simulink library "courseFollowLookAhead_cl"  (R2022a)
settings: Solver=VariableStepAuto  StartTime=0.0  StopTime=10.0  RelTol=1e-3
undefined symbols (not defined in the file or in its folder): a, pathCtrl
libraries: pathGeometry_ul x3, angleBtw2Vecs_ul x3, tanFrameProjection_ul x2, vectorNormalizer_ul x2
settings Model: Creator=James Reed  LastModifiedBy=adabney
settings SolverCC: AlgebraicLoopSolver=TrustRegion
settings DataIOCC: ReturnWorkspaceOutputs=off
settings DebuggingCC: UnconnectedInputMsg=warning  UnconnectedOutputMsg=warning  UnconnectedLineMsg=warning  SFMachineParentedDataDiag=warning  ArithmeticOperatorsInVariantConditions=warning
settings SFSimCC: CustomCodeUndefinedFunction=UseInterfaceOnly

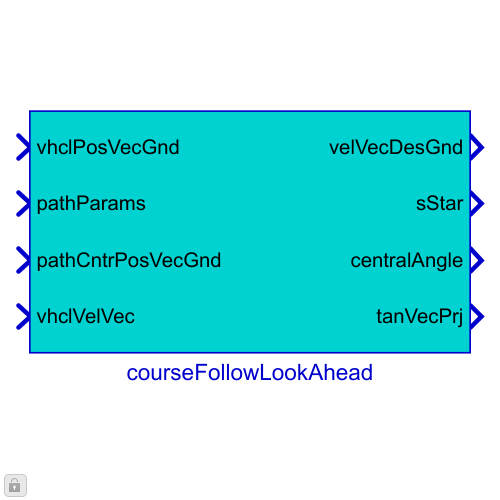
[thumbnail: Simulink's stored preview of the top-level diagram]
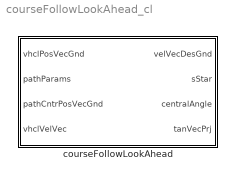
== system courseFollowLookAhead_cl ==
  courseFollowLookAhead : Subsystem

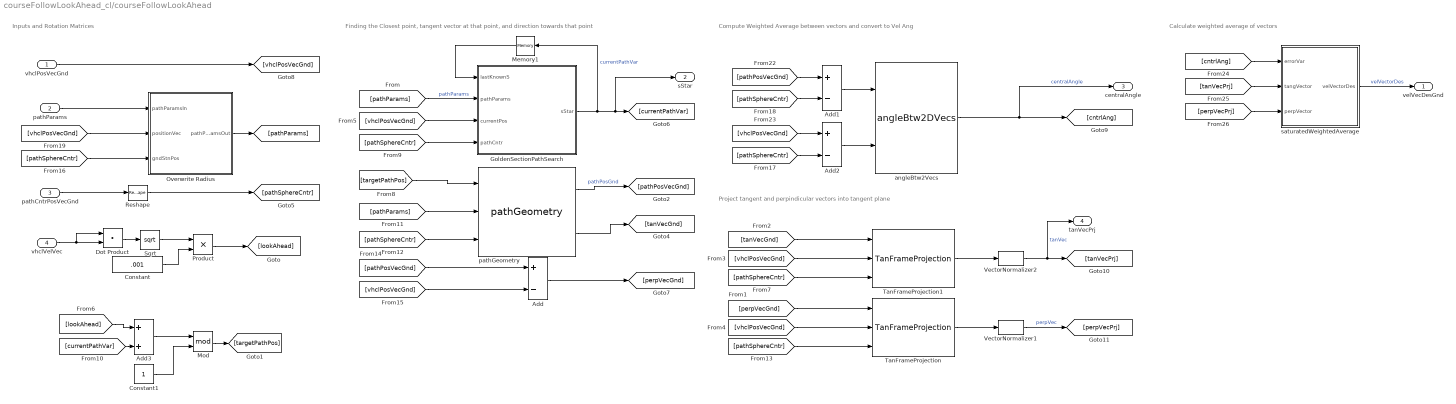
== system courseFollowLookAhead_cl/courseFollowLookAhead ==
  note: Calculate weighted average of vectors
  note: Project tangent and perpindicular vectors into tangent plane
  note: Compute Weighted Average between vectors and convert to Vel Ang
  note: Inputs and Rotation Matrices
  note: Finding the Closest point, tangent vector at that point, and direction towards that point
  "vhclPosVecGnd " : Inport
  pathParams : Inport  Port=2
  pathCntrPosVecGnd : Inport  Port=3
  vhclVelVec : Inport  Port=4
  Add : Sum  Inputs=+-
  Add1 : Sum  Inputs=+-
  Add2 : Sum  Inputs=+-
  Add3 : Sum
  Constant : Constant  Value=.001
  Constant1 : Constant
  Dot Product : DotProduct  OutDataTypeStr=Inherit: Inherit via internal rule
  GoldenSectionPathSearch : Subsystem  TreatAsAtomicUnit=on
  Memory1 : Memory  InitialCondition=pathCtrl.initPathVar.Value
  Mod : Math  Operator=mod
  Overwrite Radius : Subsystem
  Product : Product
  Reshape : Reshape  OutputDimensionality=Column vector (2-D)
  Sqrt : Sqrt
  TanFrameProjection : tanFrameProjection_ul/TanFrameProjection  SystemSampleTime=-1  VariantActivationTime=update diagram  Latency=0  AutoFrameSizeCalculation=off
  TanFrameProjection1 : tanFrameProjection_ul/TanFrameProjection  SystemSampleTime=-1  VariantActivationTime=update diagram  Latency=0  AutoFrameSizeCalculation=off
  VectorNormalizer1 : vectorNormalizer_ul/VectorNormalizer   SystemSampleTime=-1  VariantActivationTime=update diagram  Latency=0  AutoFrameSizeCalculation=off
  VectorNormalizer2 : vectorNormalizer_ul/VectorNormalizer   SystemSampleTime=-1  VariantActivationTime=update diagram  Latency=0  AutoFrameSizeCalculation=off
  angleBtw2Vecs : angleBtw2Vecs_ul/angleBtw2DVecs  SystemSampleTime=-1  VariantActivationTime=update diagram  Latency=0  AutoFrameSizeCalculation=off
  pathGeometry : pathGeometry_ul/pathGeometry  SystemSampleTime=-1  VariantActivationTime=update diagram  Latency=0  AutoFrameSizeCalculation=off
  saturatedWeightedAverage : Subsystem  mask{error_upper_lim=pathCtrl.perpErrorVal.Value}
      mask prompts: error_upper_lim "Value of Error yielding 100% perpendicular"
  velVecDesGnd : Outport  VectorParamsAs1DForOutWhenUnconnected=off
  sStar : Outport  Port=2  VectorParamsAs1DForOutWhenUnconnected=off
  centralAngle : Outport  Port=3  VectorParamsAs1DForOutWhenUnconnected=off
  tanVecPrj : Outport  Port=4
  wires:
  [pathPosVecGnd] -> Add1/1
  VectorNormalizer2/1 -> tanVecPrj/1, [tanVecPrj]  "tanVec"
  [vhclPosVecGnd] -> GoldenSectionPathSearch/3(currentPos)
  "vhclPosVecGnd "/1 -> [vhclPosVecGnd]
  pathGeometry/1 -> [pathPosVecGnd]  "pathPosGnd"
  [pathParams] -> pathGeometry/2
  VectorNormalizer1/1 -> [perpVecPrj]  "perpVec"
  angleBtw2Vecs/1 -> [cntrlAng], centralAngle/1  "centralAngle"
  [vhclPosVecGnd] -> Add2/1
  TanFrameProjection1/1 -> VectorNormalizer2/1
  [pathParams] -> GoldenSectionPathSearch/2(pathParams)  "pathParams"
  GoldenSectionPathSearch/1(sStar) -> Memory1/1, sStar/1, [currentPathVar]  "currentPathVar"
  Memory1/1 -> GoldenSectionPathSearch/1(lastKnownS)
  Add/1 -> [perpVecGnd]
  [vhclPosVecGnd] -> Add/2
  [pathPosVecGnd] -> Add/1
  pathGeometry/2 -> [tanVecGnd]
  TanFrameProjection/1 -> VectorNormalizer1/1
  Overwrite Radius/1(pathParamsOut) -> [pathParams]
  pathCntrPosVecGnd/1 -> Reshape/1
  Reshape/1 -> [pathSphereCntr]
  [pathSphereCntr] -> pathGeometry/3
  [pathSphereCntr] -> GoldenSectionPathSearch/4(pathCntr)
  [pathSphereCntr] -> Add2/2
  [pathSphereCntr] -> Add1/2
  Add1/1 -> angleBtw2Vecs/1
  Add2/1 -> angleBtw2Vecs/2
  [perpVecGnd] -> TanFrameProjection/1
  [tanVecGnd] -> TanFrameProjection1/1
  [vhclPosVecGnd] -> TanFrameProjection1/2
  [vhclPosVecGnd] -> TanFrameProjection/2
  [pathSphereCntr] -> TanFrameProjection1/3
  [pathSphereCntr] -> TanFrameProjection/3
  [cntrlAng] -> saturatedWeightedAverage/1("errorVar ")
  [tanVecPrj] -> saturatedWeightedAverage/2(tangVector)
  [perpVecPrj] -> saturatedWeightedAverage/3("perpVector ")
  saturatedWeightedAverage/1("velVectorDes ") -> velVecDesGnd/1  "velVectorDes"
  vhclVelVec/1 -> Dot Product/1, Dot Product/2
  Dot Product/1 -> Sqrt/1
  Sqrt/1 -> Product/1
  Constant/1 -> Product/2
  Product/1 -> [lookAhead]
  Add3/1 -> Mod/1
  [lookAhead] -> Add3/1
  [currentPathVar] -> Add3/2
  Constant1/1 -> Mod/2
  Mod/1 -> [targetPathPos]
  [targetPathPos] -> pathGeometry/1
  [vhclPosVecGnd] -> Overwrite Radius/2(positionVec)
  [pathSphereCntr] -> Overwrite Radius/3(gndStnPos)
  pathParams/1 -> Overwrite Radius/1(pathParamsIn)

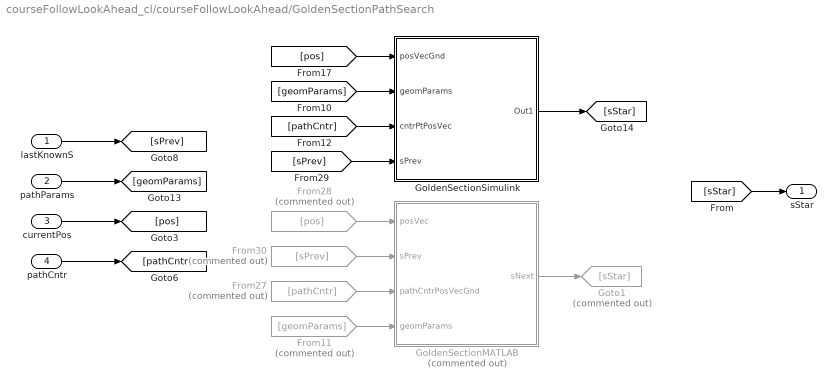
== system courseFollowLookAhead_cl/courseFollowLookAhead/GoldenSectionPathSearch ==
  lastKnownS : Inport
  pathParams : Inport  Port=2
  currentPos : Inport  Port=3
  pathCntr : Inport  Port=4
  From11 : From  Commented=on  GotoTag=geomParams
  From27 : From  Commented=on  GotoTag=pathCntr
  From28 : From  Commented=on  GotoTag=pos
  From30 : From  Commented=on  GotoTag=sPrev
  GoldenSectionMATLAB : MATLAB Function  Commented=on  TreatAsAtomicUnit=on  mask{geomFunc=pathCtrl, searchWidth=0.1, pathVarTol=1e-5}
  GoldenSectionSimulink : Subsystem
  Goto1 : Goto  Commented=on  GotoTag=sStar
  sStar : Outport  InitialOutput=pathCtrl.initPathVar.Value  VectorParamsAs1DForOutWhenUnconnected=off
  wires:
  currentPos/1 -> [pos]
  pathParams/1 -> [geomParams]
  pathCntr/1 -> [pathCntr]
  GoldenSectionMATLAB/1(sNext) -> Goto1/1
  From11/1 -> GoldenSectionMATLAB/4(geomParams)
  From28/1 -> GoldenSectionMATLAB/1(posVec)
  From30/1 -> GoldenSectionMATLAB/2(sPrev)
  From27/1 -> GoldenSectionMATLAB/3(pathCntrPosVecGnd)
  lastKnownS/1 -> [sPrev]
  [sStar] -> sStar/1
  [pos] -> GoldenSectionSimulink/1(posVecGnd)
  [geomParams] -> GoldenSectionSimulink/2(geomParams)
  [pathCntr] -> GoldenSectionSimulink/3(cntrPtPosVec)
  [sPrev] -> GoldenSectionSimulink/4(sPrev)
  GoldenSectionSimulink/1(Out1) -> [sStar]

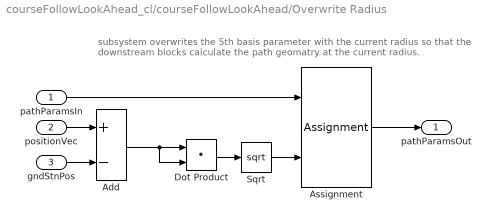
== system courseFollowLookAhead_cl/courseFollowLookAhead/Overwrite Radius ==
  note: subsystem overwrites the 5th basis parameter with the current radius
      | so that the downstream blocks calculate the path geomatry at the current radius.
  pathParamsIn : Inport
  positionVec : Inport  Port=2
  gndStnPos : Inport  Port=3
  Add : Sum  Inputs=+-
  Assignment : Assignment  NumberOfDimensions=2  DiagnosticForDimensions=Warning  IndexOptions=Index vector (dialog),Assign all  Indices=5,5  OutputSizes=1,1
  Dot Product : DotProduct  OutDataTypeStr=Inherit: Inherit via internal rule
  Sqrt : Sqrt
  pathParamsOut : Outport  VectorParamsAs1DForOutWhenUnconnected=off
  wires:
  Add/1 -> Dot Product/2, Dot Product/1
  Dot Product/1 -> Sqrt/1
  Assignment/1 -> pathParamsOut/1
  Sqrt/1 -> Assignment/2
  pathParamsIn/1 -> Assignment/1
  positionVec/1 -> Add/1
  gndStnPos/1 -> Add/2

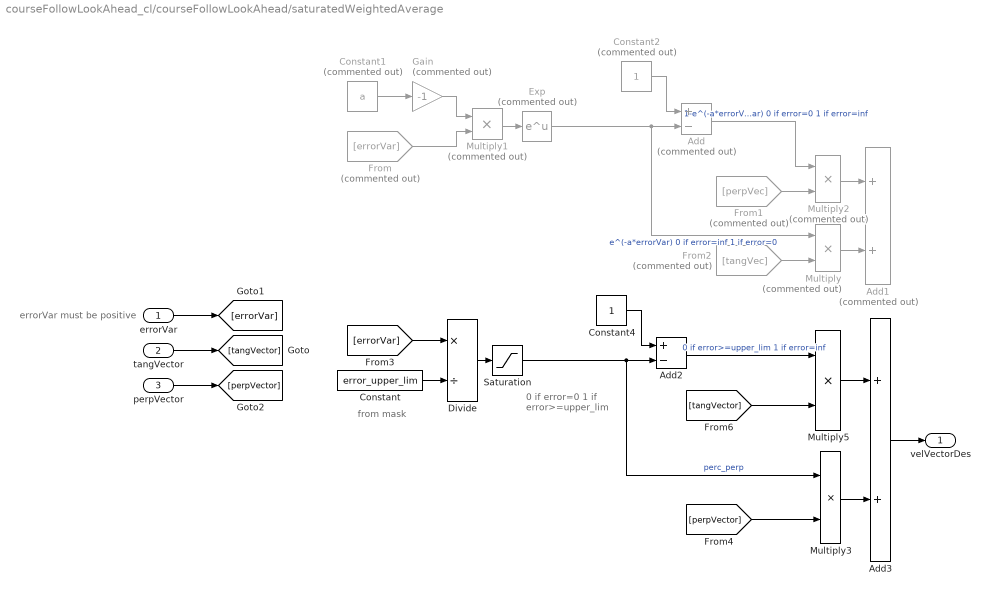
== system courseFollowLookAhead_cl/courseFollowLookAhead/saturatedWeightedAverage ==
  note: errorVar must be positive
  note: from mask
  note: 0 if error=0
      | 1 if error>=upper_lim
  "errorVar " : Inport
  tangVector : Inport  Port=2
  "perpVector " : Inport  Port=3
  Add : Sum  Commented=on  Inputs=+-
  Add1 : Sum  Commented=on
  Add2 : Sum  Inputs=+-
  Add3 : Sum
  Constant : Constant  Value=error_upper_lim
  Constant1 : Constant  Commented=on  Value=a
  Constant2 : Constant  Commented=on
  Constant4 : Constant
  Divide : Product  Inputs=*/
  Exp : Math  Commented=on  SignedPower=on
  From : From  Commented=on  GotoTag=errorVar
  From1 : From  Commented=on  GotoTag=perpVec
  From2 : From  Commented=on  GotoTag=tangVec
  Gain : Gain  Commented=on  Gain=-1
  Multiply : Product  Commented=on
  Multiply1 : Product  Commented=on
  Multiply2 : Product  Commented=on
  Multiply3 : Product
  Multiply5 : Product
  Saturation : Saturate  UpperLimit=1  LowerLimit=0
  "velVectorDes " : Outport  VectorParamsAs1DForOutWhenUnconnected=off
  wires:
  [perpVector] -> Multiply3/2
  [tangVector] -> Multiply5/2
  Divide/1 -> Saturation/1
  Constant/1 -> Divide/2
  [errorVar] -> Divide/1
  Add2/1 -> Multiply5/1  "0 if error>=upper_lim 1 if error=inf"
  Multiply5/1 -> Add3/1
  Multiply3/1 -> Add3/2
  Add3/1 -> "velVectorDes "/1
  Saturation/1 -> Add2/2, Multiply3/1  "perc_perp"
  Constant4/1 -> Add2/1
  From2/1 -> Multiply/2
  From1/1 -> Multiply2/2
  Multiply/1 -> Add1/2
  Multiply2/1 -> Add1/1
  From/1 -> Multiply1/2
  "perpVector "/1 -> [perpVector]
  "errorVar "/1 -> [errorVar]
  Add/1 -> Multiply2/1  "1-e^(-a*errorVar) 0 if error=0 1 if error=inf"
  Constant2/1 -> Add/1
  Exp/1 -> Add/2, Multiply/1  "e^(-a*errorVar) 0 if error=inf 1 if error=0"
  Multiply1/1 -> Exp/1
  Gain/1 -> Multiply1/1
  Constant1/1 -> Gain/1
  tangVector/1 -> [tangVector]

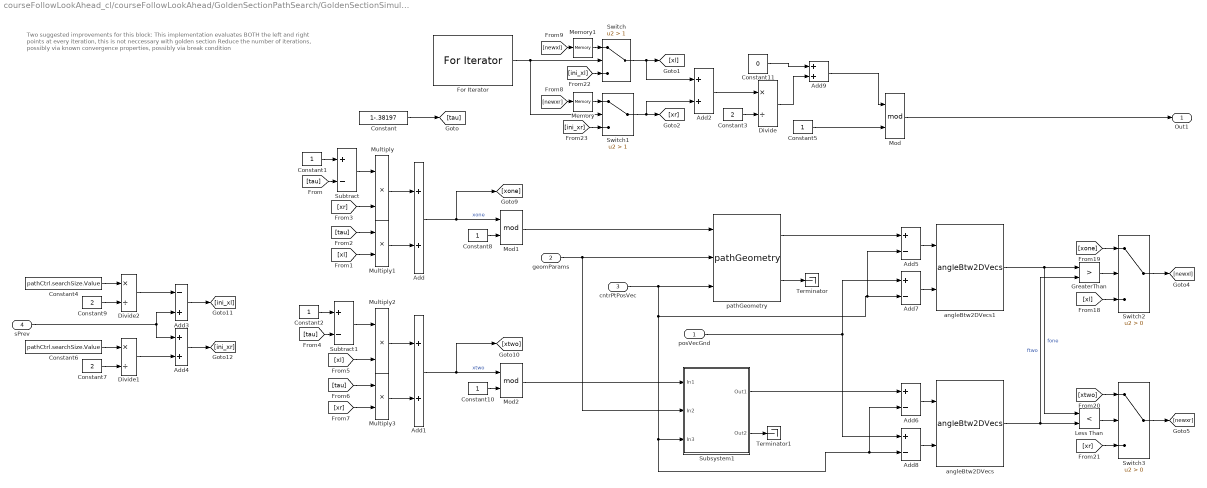
== system courseFollowLookAhead_cl/courseFollowLookAhead/GoldenSectionPathSearch/GoldenSectionSimulink ==
  note: Two suggested improvements for this block:
      | This implementation evaluates BOTH the left and right points at every iteration, this is not neccessary with golden section
      | Reduce the number of iterations, possibly via known convergence properties, possibly via break condition
  posVecGnd : Inport
  geomParams : Inport  Port=2
  cntrPtPosVec : Inport  Port=3
  sPrev : Inport  Port=4
  Add{,1..2,4,9} (5 alike) : Sum
  Add3 : Sum  Inputs=-+
  Add{5..8} (4 alike) : Sum  Inputs=+-
  Constant : Constant  Value=1-.38197
  Constant{1..2,5,8,10} (5 alike) : Constant
  Constant11 : Constant  Value=0
  Constant3 : Constant  Value=2
  Constant4 : Constant  Value=pathCtrl.searchSize.Value
  Constant6 : Constant  Value=pathCtrl.searchSize.Value
  Constant7 : Constant  Value=2
  Constant9 : Constant  Value=2
  Divide : Product  Inputs=*/
  Divide1 : Product  Inputs=*/
  Divide2 : Product  Inputs=*/
  For Iterator : ForIterator  IterationLimit=25
  GreaterThan : RelationalOperator  Operator=>  OutDataTypeStr=boolean  RndMeth=Simplest  InputSameDT=off
  Less Than : RelationalOperator  Operator=<  OutDataTypeStr=boolean  RndMeth=Simplest  InputSameDT=off
  Memory : Memory  InheritSampleTime=on
  Memory1 : Memory  InheritSampleTime=on
  Mod : Math  Operator=mod  SignedPower=on
  Mod1 : Math  Operator=mod  SignedPower=on
  Mod2 : Math  Operator=mod  SignedPower=on
  Multiply{,1..3} (4 alike) : Product
  Subsystem1 : Subsystem
  Subtract : Sum  Inputs=+-
  Subtract1 : Sum  Inputs=+-
  Switch : Switch  Criteria=u2 > Threshold  Threshold=1  SaturateOnIntegerOverflow=off  InputSameDT=off
  Switch1 : Switch  Criteria=u2 > Threshold  Threshold=1  SaturateOnIntegerOverflow=off  InputSameDT=off
  Switch2 : Switch  Criteria=u2 > Threshold  SaturateOnIntegerOverflow=off  InputSameDT=off
  Switch3 : Switch  Criteria=u2 > Threshold  SaturateOnIntegerOverflow=off  InputSameDT=off
  Terminator : Terminator
  Terminator1 : Terminator
  angleBtw2DVecs : angleBtw2Vecs_ul/angleBtw2DVecs  SystemSampleTime=-1  VariantActivationTime=update diagram  Latency=0  AutoFrameSizeCalculation=off
  angleBtw2DVecs1 : angleBtw2Vecs_ul/angleBtw2DVecs  SystemSampleTime=-1  VariantActivationTime=update diagram  Latency=0  AutoFrameSizeCalculation=off
  pathGeometry : pathGeometry_ul/pathGeometry  SystemSampleTime=-1  VariantActivationTime=update diagram  Latency=0  AutoFrameSizeCalculation=off
  Out1 : Outport
  wires:
  Subtract1/1 -> Multiply2/1
  cntrPtPosVec/1 -> Add6/2, Add8/2, Subsystem1/3(In3), Add5/2, Add7/2, pathGeometry/3
  Switch/1 -> Add2/1, [xl]
  geomParams/1 -> pathGeometry/2, Subsystem1/2(In2)
  Constant2/1 -> Subtract1/1
  Subsystem1/1(Out1) -> Add6/1
  [xr] -> Multiply3/2
  Constant8/1 -> Mod1/2
  pathGeometry/1 -> Add5/1
  GreaterThan/1 -> Switch2/2
  posVecGnd/1 -> Add8/1, Add7/1
  Constant1/1 -> Subtract/1
  Constant5/1 -> Mod/2
  angleBtw2DVecs/1 -> GreaterThan/2, Less Than/2  "ftwo"
  [tau] -> Subtract1/2
  Add1/1 -> [xtwo], Mod2/1  "xtwo"
  Constant7/1 -> Divide1/2
  Subtract/1 -> Multiply/1
  Subsystem1/2(Out2) -> Terminator1/1
  [xl] -> Multiply1/2
  Multiply/1 -> Add/1
  [xtwo] -> Switch3/1
  [tau] -> Subtract/2
  [tau] -> Multiply3/1
  Memory1/1 -> Switch/1
  For Iterator/1 -> Switch1/2, Switch/2
  Add/1 -> [xone], Mod1/1  "xone"
  Constant/1 -> [tau]
  Switch1/1 -> Add2/2, [xr]
  Multiply2/1 -> Add1/1
  Mod2/1 -> Subsystem1/1(In1)
  Constant4/1 -> Divide2/1
  angleBtw2DVecs1/1 -> Less Than/1, GreaterThan/1  "fone"
  [ini_xr] -> Switch1/3
  [xone] -> Switch2/1
  [tau] -> Multiply1/1
  Add7/1 -> angleBtw2DVecs1/2
  [newxr] -> Memory/1
  Memory/1 -> Switch1/1
  Mod1/1 -> pathGeometry/1
  Divide1/1 -> Add4/2
  Add3/1 -> [ini_xl]
  [xr] -> Multiply/2
  Constant9/1 -> Divide2/2
  Add4/1 -> [ini_xr]
  Constant3/1 -> Divide/2
  Less Than/1 -> Switch3/2
  sPrev/1 -> Add4/1, Add3/2
  Add5/1 -> angleBtw2DVecs1/1
  Multiply3/1 -> Add1/2
  [xl] -> Multiply2/2
  [xr] -> Switch3/3
  [xl] -> Switch2/3
  Add2/1 -> Divide/1
  Constant10/1 -> Mod2/2
  Add6/1 -> angleBtw2DVecs/1
  Constant6/1 -> Divide1/1
  [newxl] -> Memory1/1
  pathGeometry/2 -> Terminator/1
  Switch2/1 -> [newxl]
  Divide2/1 -> Add3/1
  Mod/1 -> Out1/1
  [ini_xl] -> Switch/3
  Switch3/1 -> [newxr]
  Multiply1/1 -> Add/2
  Add8/1 -> angleBtw2DVecs/2
  Divide/1 -> Add9/2
  Add9/1 -> Mod/1
  Constant11/1 -> Add9/1

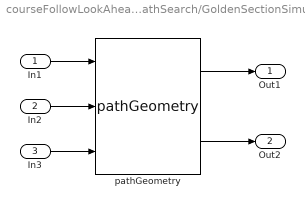
== system courseFollowLookAhead_cl/courseFollowLookAhead/GoldenSectionPathSearch/GoldenSectionSimulink/Subsystem1 ==
  In1 : Inport
  In2 : Inport  Port=2
  In3 : Inport  Port=3
  pathGeometry : pathGeometry_ul/pathGeometry  SystemSampleTime=-1  VariantActivationTime=update diagram  Latency=0  AutoFrameSizeCalculation=off
  Out1 : Outport  VectorParamsAs1DForOutWhenUnconnected=off
  Out2 : Outport  Port=2  VectorParamsAs1DForOutWhenUnconnected=off
  wires:
  In2/1 -> pathGeometry/2
  pathGeometry/1 -> Out1/1
  In3/1 -> pathGeometry/3
  In1/1 -> pathGeometry/1
  pathGeometry/2 -> Out2/1

== matlab function courseFollowLookAhead_cl/courseFollowLookAhead/GoldenSectionPathSearch/GoldenSectionMATLAB ==
  data: posVec input; sNext output; sPrev input; pathCntrPosVecGnd input; pathVarTol parameter; searchWidth parameter; geomParams input
function sNext = fcn(posVec,sPrev,pathCntrPosVecGnd, pathVarTol, searchWidth, geomParams)
% I wrote this function on 4/22/2020 when attempting to figure out some
% issues with numerical stiffness.  Turns out that althought the profiler
% was telling me the problem was with the simulink in the equivalent
% subsystem, that was a lie.  Anyways, I thought I should leave this here
% anyways just in case anyone wants to reference it.  Note that this
% implementation doesn't allow for different paths without changing
% function J below.  Which isn't great for a long term solution, so don't
% just use this as-is if you want to go to a matlab-based golden section
% implementation in the future. Also, I think there are some hard-coded
% numbers in the mask in the model, so fix that.  Finally, note that even
% though the "equivalent" simulink implementation has some inefficiencies
% that this code doesnt (as noted in the simulink implementation), there
% doesn't appear to be a siginificant difference in run times, although I
% haven't done a thorough study. -Mitchell

% phi = (sqrt(5) + 1) / 2;
% gr = 1/((1/phi)+1);
% gr = 0.618033988749895;
x1 = sPrev - searchWidth/2;
x4 = sPrev + searchWidth/2;
x2 = x4 - (x4-x1)*0.618033988749895;
x3 = x1 + (x4-x1)*0.618033988749895;
% J1 = J(x1,posVec,geomParams,pathCntrPosVecGnd);
J2 = J(x2,posVec,geomParams,pathCntrPosVecGnd);
J3 = J(x3,posVec,geomParams,pathCntrPosVecGnd);
% J4 = J(x4,posVec,geomParams,pathCntrPosVecGnd);
% JL =JFunc(xL);
% JR = JFunc(xR);
% plot([x1 x2 x3 x4],[J1 J2 J3 J4])
for ii = 1:100 
    if J2<J3
        x4 = x3;
%         J4 = J(x4,posVec,geomParams,pathCntrPosVecGnd);
        x3 = x2;
        J3 = J2;
        x2 = x4 - (x4-x1)*0.618033988749895;
        J2 = J(x2,posVec,geomParams,pathCntrPosVecGnd);
    else
        x1 = x2;
%         J1 = J(x1,posVec,geomParams,pathCntrPosVecGnd);
        x2 = x3;
        J2 = J3;
        x3 = x1 + (x4-x1)*0.618033988749895;
        J3 = J(x3,posVec,geomParams,pathCntrPosVecGnd);
    end
    if x4-x1<pathVarTol/2
        break
    end
end
sNext = mod((x4+x1)/2,1);
end

function val = J(sTest,posVec,geomParams,pathCntr)
az = atan2(posVec(2),posVec(1));
el = atan2(posVec(3),sqrt(posVec(1)^2+posVec(2)^2));
pathPosVec = lemOfBooth(sTest,geomParams,pathCntr);
azP = atan2(pathPosVec(2),pathPosVec(1));
elP = atan2(pathPosVec(3),sqrt(pathPosVec(1)^2+pathPosVec(2)^2));
val = (az-azP)^2+(el-elP)^2;
end
